simulink model "dspsdadc_fixpt"  (Simulink 6.0)
settings: Solver=ode5  SolverMode=SingleTasking  StartTime=0.0  StopTime=inf  FixedStep=1/(512*1024)  MaxStep=1/512000  RelTol=1e-3  AbsTol=1e-6
libraries: dspmlti3 x3, dspddes2 x1, dspbuff3 x1, dspmlti4 x1
settings Model: Creator=don  LastModifiedBy=sconahan  ExtModeTrigMode=oneshot  ExtModeArmWhenConnect=off  ExtModeAutoUpdateStatusClock=off
settings DataIOCC: LimitDataPoints=off  SaveOutput=off  SaveTime=off  SignalLoggingName=logsOut
settings OptimizationCC: BlockReduction=off  BooleanDataType=off  MultiInstanced=off  RollThreshold=2
settings FormatCC: IgnoreBidirectionalLines=off
settings DebuggingCC: IntegerOverflowMsg=none  ParameterPrecisionLossMsg=none
settings HardwareCC: TargetUnknown=on
settings CodeAppCC: FileBanners=off  CustomSymbols=off
settings GRTTargetCC: TargetFcnLib=iso_c_tmw.mat  IsERTTarget=off

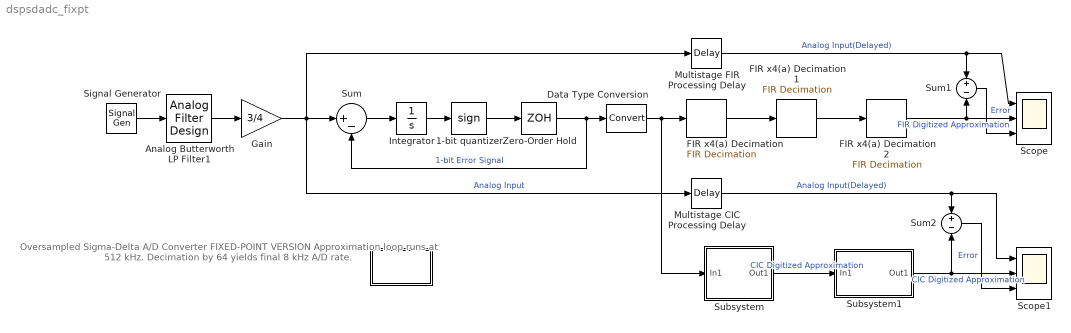
== system dspsdadc_fixpt ==
  note: Oversampled Sigma-Delta A/D Converter
      | FIXED-POINT VERSION
      | Approximation loop runs at 512 kHz.
      | Decimation by 64 yields final 8 kHz A/D rate.
  " " : Subsystem
      mask Type: Sigma-delta demo Info block
      mask Display: disp('Info')
  1-bit quantizer : Signum
  Analog Butterworth LP Filter1 : dspddes2/Analog Filter Design  method=Butterworth  filttype=Lowpass  N=5  Wlo=2*pi*400  Whi=80  Rp=3  Rs=40
  Data Type Conversion : DataTypeConversion  OutDataTypeMode=Specify via dialog  OutDataType=sfix(2)
  FIR x4(a) Decimation : dspmlti3/FIR Decimation  h=fir1(31,0.15)  D=4  framing=Maintain input frame size  outputBufInitCond=0  firstCoeffMode=Binary point scaling  firstCoeffWordLength=16  firstCoeffFracLength=15  prodOutputMode=Binary point scaling  prodOutputWordLength=16  prodOutputFracLength=14  roundingMode=Floor  overflowMode=off
      settings: additionalParams=on
  FIR x4(a) Decimation1 : dspmlti3/FIR Decimation  h=fir1(31,0.15)  D=4  framing=Maintain input frame size  outputBufInitCond=0  firstCoeffMode=Binary point scaling  firstCoeffWordLength=16  firstCoeffFracLength=15  prodOutputMode=Binary point scaling  prodOutputWordLength=16  prodOutputFracLength=14  roundingMode=Floor  overflowMode=off
      settings: additionalParams=on
  FIR x4(a) Decimation2 : dspmlti3/FIR Decimation  h=fir1(31,0.15)  D=4  framing=Maintain input frame size  outputBufInitCond=0  firstCoeffMode=Binary point scaling  firstCoeffWordLength=16  firstCoeffFracLength=15  prodOutputMode=Binary point scaling  prodOutputWordLength=16  prodOutputFracLength=14  roundingMode=Floor  overflowMode=off
      settings: additionalParams=on
  Gain : Gain  Gain=3/4  SaturateOnIntegerOverflow=on
  Integrator : Integrator
  Multistage CIC Processing Delay : TransportDelay  DelayTime=250/512000
  Multistage FIR Processing Delay : TransportDelay  DelayTime=357/512000
  Scope : Scope  NumInputPorts=3
      settings: TimeRange=0.025  YMin=-1.1~-1.1~-0.25  YMax=1.1~1.1~0.25
  Scope1 : Scope  NumInputPorts=3
      settings: TimeRange=0.025  YMin=-1.1~-1.1~-0.25  YMax=1.1~1.1~0.25
  Signal Generator : SignalGenerator  WaveForm=square  Frequency=80
  Subsystem : Subsystem
      mask Display: disp('CIC\nDecimation\nFilter')
  Subsystem1 : Subsystem
      mask Display: disp('Rescaling for\nComparison')
  Sum : Sum  Inputs=|+-  SaturateOnIntegerOverflow=on  InputSameDT=on
  Sum1 : Sum  Inputs=+-  RndMeth=Nearest  SaturateOnIntegerOverflow=on
  Sum2 : Sum  Inputs=+-  RndMeth=Nearest  SaturateOnIntegerOverflow=on
  Zero-Order Hold : ZeroOrderHold  SampleTime=1/(512*1024)
  wires:
  Zero-Order Hold/1 -> Data Type Conversion/1, Sum/2  "1-bit Error Signal"
  1-bit quantizer/1 -> Zero-Order Hold/1
  Sum/1 -> Integrator/1
  Integrator/1 -> 1-bit quantizer/1
  FIR x4(a) Decimation2/1 -> Scope/2, Sum1/2  "FIR Digitized Approximation"
  Gain/1 -> Sum/1, Multistage FIR Processing Delay/1, Multistage CIC Processing Delay/1  "Analog Input"
  Analog Butterworth LP Filter1/1 -> Gain/1
  Signal Generator/1 -> Analog Butterworth LP Filter1/1
  FIR x4(a) Decimation/1 -> FIR x4(a) Decimation1/1
  FIR x4(a) Decimation1/1 -> FIR x4(a) Decimation2/1
  Sum1/1 -> Scope/3  "Error"
  Multistage FIR Processing Delay/1 -> Sum1/1, Scope/1  "Analog Input(Delayed)"
  Data Type Conversion/1 -> FIR x4(a) Decimation/1, Subsystem/1(In1)
  Subsystem/1(Out1) -> Subsystem1/1(In1)  "CIC Digitized Approximation"
  Sum2/1 -> Scope1/3  "Error"
  Multistage CIC Processing Delay/1 -> Sum2/1, Scope1/1  "Analog Input(Delayed)"
  Subsystem1/1(Out1) -> Sum2/2, Scope1/2  "CIC Digitized Approximation"

== system dspsdadc_fixpt/  ==
  note: Oversampled Sigma-Delta A/D Converter
      |
      | The Oversampled Sigma-Delta A/D Converter is a noise-shaping quantizer.  The main purpose of
      | noise-shaping is to reshape the spectrum of quantization noise so that most of the noise is filtered
      |  out of the relevant frequency band (say the audio band for speech applications).
      |
      | The main objective here is to trade off bits for samples - that is, increasing the sampling rate but
      | reducing the number of bits per sample. The resulting increase in quantization noise is compensated
      |  by a noise shaping quantizer.  This quantizer pushes the added quantization noise out of the relevant
      | frequency band and thereby preserves a desired level of signal quality. This reduction in the number
      | of bits simplifies the structure of A/D and D/A converters.
      |
      | As seen in the demo, the analog input is prefiltered by an antialiasing prefilter whose structure is
      |  simplified (order 5) because of oversampling. The input signal is oversampled by a factor of 64 and
      |  a two-level ADC (1-bit quantizer) is used. The Zero-Order Hold converts it back to analog form, which
      | is then subtracted from the analog input. The difference signal, which is the "delta" part, is accumulated
      | into the integrator, which is the "sigma" part, and provides a local average of the input. The feedback
      |  loop (approximation loop) causes the quantization noise generated by the ADC to be highpass filtered,
      |  pushing its energy towards the higher frequencies (64*fs/2) and away from the relevant signal band.
      |
      | The multistage decimation stage (4*4*4) reduces the sampling rate back to 8 KHz. During this process,
      |  it removes the high frequency quantization noise that was introduced by the feedback loop and
      |  removes any undesired frequency components beyond fs/2 (4 KHz) that were not removed by the
      | simple analog prefilter,
      |
      | For more information on the 'Oversampled Sigma-Delta A/D Convertor', see S. J. Orfanidis,
      | "Introduction To Signal Processing", Prentice Hall, 1996.

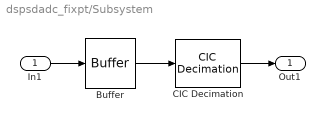
== system dspsdadc_fixpt/Subsystem ==
  In1 : Inport
  Buffer : dspbuff3/Buffer  N=64  V=0  ic=0
  CIC Decimation : dspmlti4/CIC Decimation  filtFrom=Dialog  filtobj=Hm_decim  ftype=Zero-latency decimator  R=64  resampPhase=0  M=1  N=5  BPS=[32 30 24 20 16 16 16 16 16 16]  launchFVT=off  framing=Maintain input frame rate
  Out1 : Outport
  wires:
  CIC Decimation/1 -> Out1/1
  Buffer/1 -> CIC Decimation/1
  In1/1 -> Buffer/1

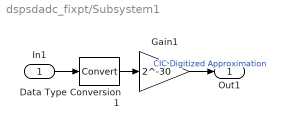
== system dspsdadc_fixpt/Subsystem1 ==
  In1 : Inport
  Data Type Conversion1 : DataTypeConversion  OutDataTypeMode=single  OutDataType=sfix(2)
  Gain1 : Gain  Gain=2^-30  SaturateOnIntegerOverflow=on
  Out1 : Outport
  wires:
  Data Type Conversion1/1 -> Gain1/1
  In1/1 -> Data Type Conversion1/1
  Gain1/1 -> Out1/1  "CIC Digitized Approximation"
